simulink model "Referentiel"  (R2020b)
settings: Solver=FixedStepAuto  StartTime=0.0  StopTime=inf  FixedStep=0.05  RelTol=1e-3
model workspace: external: MATLAB File C:\Users\antoi\OneDrive\Desktop\Matlab-Simulink\Test Robotique\Bras_DataFile.m (data not in the file)
undefined symbols (not defined in the file): X, Y, Z
libraries: robotlib x4, robotmaniplib x1
settings Model: SimulationMode=external  PacingRate=0.050000  Creator=antoi  LastModifiedBy=alessandrini
settings OptimizationCC: EnhancedBackFolding=on  PassReuseOutputArgsAs=Individual arguments  ZeroExternalMemoryAtStartup=off  ZeroInternalMemoryAtStartup=off  MaxStackSize=64  OptimizeBlockOrder=speed  DifferentSizesBufferReuse=on  OptimizationCustomize=off  EfficientTunableParamExpr=on
settings DebuggingCC: ParameterTunabilityLossMsg=error
settings HardwareCC: ProdBitPerPointer=32  ProdBitPerSizeT=32  ProdBitPerPtrDiffT=32  ProdLargestAtomicFloat=None  ProdIntDivRoundTo=Undefined  ProdEndianess=Unspecified  ProdWordSize=32  ProdHWDeviceType=Generic->Unspecified (assume 32-bit Generic)  UseEmbeddedCoderFeatures=off
settings RTWCC: Description=Embedded Coder  SystemTargetFile=ert.tlc  HardwareBoard=Robot Operating System (ROS)  TLCOptions="-aInlineSetEventsForThisBaseRateFcn=TLC_FALSE -aSuppressMultiTaskScheduler=TLC_FALSE  -aRateBasedStepFcn=0"  TemplateMakefile=ert_default_tmf  GenerateReport=on  Toolchain=Catkin  LaunchReport=on  TargetLang=C++
settings CodeAppCC: ForceParamTrailComments=on  OperatorAnnotations=on  SimulinkDataObjDesc=on  SFDataObjDesc=on  InsertBlockDesc=on
settings ERTTargetCC: SupportNonInlinedSFcns=on  ExtMode=on  ExtModeMexArgs='127.0.0.1' 0 17725  ERTSrcFileBannerTemplate=codertarget_code_template.cgt  ERTHdrFileBannerTemplate=codertarget_code_template.cgt  ERTDataSrcFileTemplate=codertarget_code_template.cgt  ERTDataHdrFileTemplate=codertarget_code_template.cgt

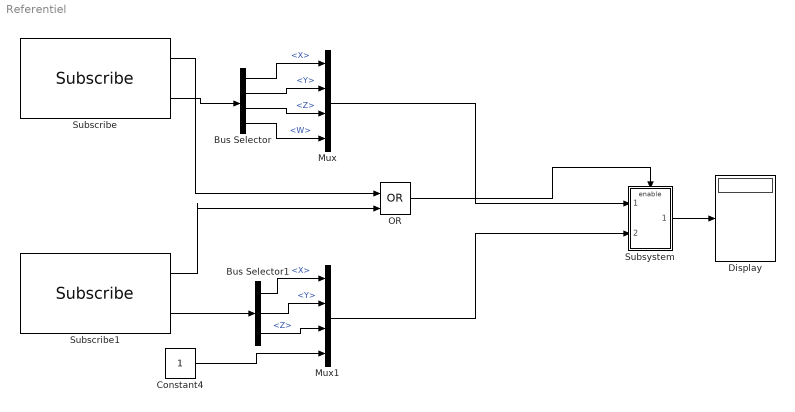
== system Referentiel ==
  Bus Selector : BusSelector  OutputSignals=X,Y,Z,W
  Bus Selector1 : BusSelector  OutputSignals=X,Y,Z
  Constant4 : Constant
  Display : Display
  Mux : Mux
  Mux1 : Mux
  OR : Logic  Operator=OR  IconShape=distinctive  AllPortsSameDT=off  OutDataTypeStr=boolean
  Subscribe : robotlib/Subscribe  topicSource=Specify your own  topic=/angles_referentiel  messageType=geometry_msgs/Quaternion  SampleTime=-1  legacyBusStruct=off  messageQueueLength=1
  Subscribe1 : robotlib/Subscribe  topicSource=Specify your own  topic=/position_camera  messageType=geometry_msgs/Point  SampleTime=-1  legacyBusStruct=off  messageQueueLength=1
  Subsystem : Subsystem
  wires:
  Bus Selector1/1 -> Mux1/1  "<X>"
  Bus Selector1/2 -> Mux1/2  "<Y>"
  Subscribe1/2 -> Bus Selector1/1
  Bus Selector1/3 -> Mux1/3  "<Z>"
  Constant4/1 -> Mux1/4
  Subscribe/2 -> Bus Selector/1
  Bus Selector/1 -> Mux/1  "<X>"
  Bus Selector/2 -> Mux/2  "<Y>"
  Bus Selector/3 -> Mux/3  "<Z>"
  Bus Selector/4 -> Mux/4  "<W>"
  Subscribe1/1 -> OR/2
  Subscribe/1 -> OR/1
  Mux/1 -> Subsystem/1(Config)
  Mux1/1 -> Subsystem/2(In2)
  OR/1 -> Subsystem/Enable
  Subsystem/1(Out1) -> Display/1

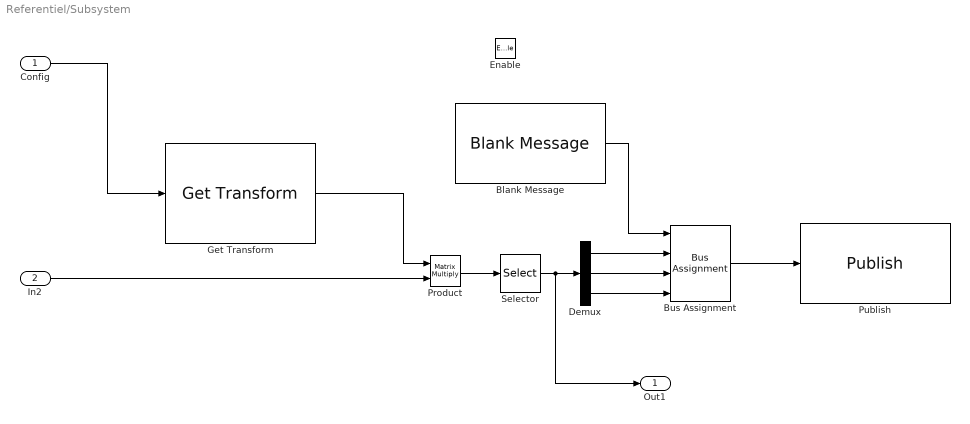
== system Referentiel/Subsystem ==
  Config : Inport
  In2 : Inport  Port=2
  Enable : EnablePort
  Blank Message : robotlib/Blank Message  messageClass=Message  entityType=geometry_msgs/Point  messageType=geometry_msgs/Point  SampleTime=0.05  legacyBusStruct=off
  Bus Assignment : BusAssignment  AssignedSignals=X,Y,Z
  Demux : Demux  Outputs=3
  Get Transform : robotmaniplib/Get Transform  RigidBodyTree=robot  SourceBody=Body6  TargetBody=Base  SimulateUsing=Interpreted execution
  Product : Product  Multiplication=Matrix(*)
  Publish : robotlib/Publish  topicSource=Specify your own  topic=/position_robot  messageType=geometry_msgs/Point  legacyBusStruct=off  messageQueueLength=1
  Selector : Selector  InputPortWidth=4  IndexOptions=Starting index (dialog)  Indices=[1]  OutputSizes=3
  Out1 : Outport
  wires:
  Selector/1 -> Out1/1, Demux/1
  In2/1 -> Product/2
  Blank Message/1 -> Bus Assignment/1
  Product/1 -> Selector/1
  Bus Assignment/1 -> Publish/1
  Config/1 -> Get Transform/1
  Get Transform/1 -> Product/1
  Demux/1 -> Bus Assignment/2
  Demux/3 -> Bus Assignment/4
  Demux/2 -> Bus Assignment/3
